simulink model "tankTry2"  (R2020a)
settings: Solver=VariableStepAuto  StartTime=0.0  StopTime=500  RelTol=1e-3
libraries: mpclib x1, simulink x1
settings Model: Creator=lydialagorga  LastModifiedBy=lydialagorga

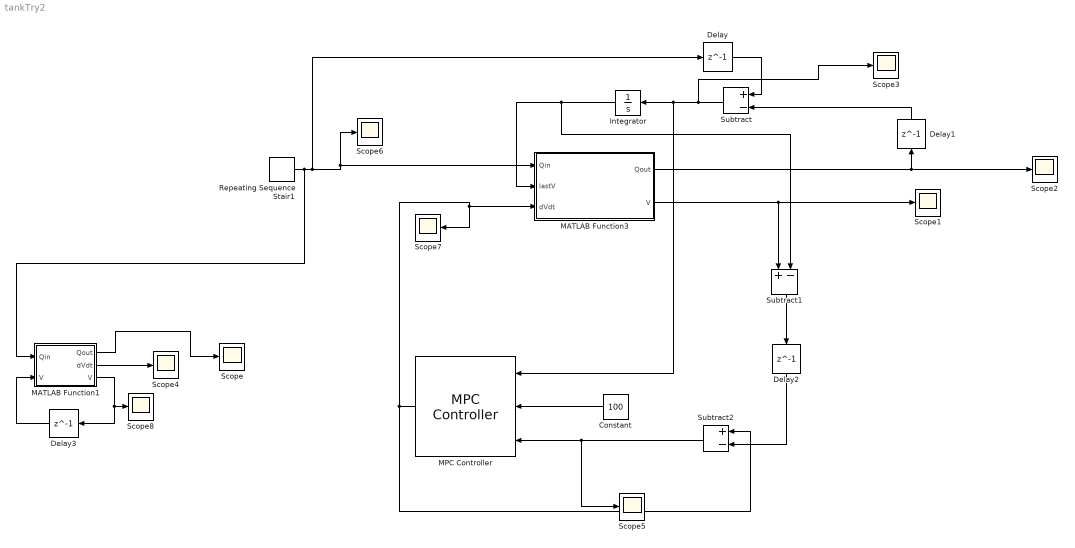
== system tankTry2 ==
  Constant : Constant  Value=100
  Delay{,1..3} (4 alike) : Delay  DelayLength=1  InitialCondition=0
  Integrator : Integrator
  MATLAB Function1 : MATLAB Function  TreatAsAtomicUnit=on
  MATLAB Function3 : MATLAB Function  TreatAsAtomicUnit=on
  MPC Controller : mpclib/MPC Controller  SCDEnableBlockLinearizationSpecification=on  mpcobj=MPCobj  is_multiple=0  enable_value=0  return_u0=off  updateMPCinCallerWorkspace=on  md_inport=on  mv_inport=off  uref_inport=off  return_cost=off  return_mvseq=off  return_qpstatus=off  return_xseq=off  return_state=off  return_ovseq=off  state_inport=off  umin_inport=off  umax_inport=off  ymin_inport=off  ymax_inport=off  cc_inport=off  ywt_inport=off  uwt_inport=off  duwt_inport=off  rhoeps_inport=off  pm_inport=off  MaximumP=10  HorizonChoice=FixedHorizon  n_ts=1  n_p=10  n_mv=1  n_md=1  n_ud=0  n_mo=1  n_uo=0  BlockDataType=double  SampleTimeInherited=off  switch_inport=off
  Repeating Sequence Stair1 : simulink/Sources/Repeating Sequence Stair  OutValues=[3 1 4 2 1]  tsamp=-1  OutMin=[]  OutMax=[]  OutDataTypeStr=double  OutputDataTypeScalingMode=double  OutDataType=fixdt(0,8)  ConRadixGroup=Best Precision: Vector-wise  OutScaling=2^-12
  Scope{,1..8} (9 alike) : Scope
  Subtract : Sum  Inputs=+-
  Subtract1 : Sum  Inputs=+-
  Subtract2 : Sum  Inputs=+-
  wires:
  MPC Controller/1 -> Scope7/1, MATLAB Function3/3(dVdt), Subtract2/1
  Repeating Sequence Stair1/1 -> MATLAB Function1/1(Qin), Delay/1, MATLAB Function3/1(Qin), Scope6/1
  Delay/1 -> Subtract/1
  Delay1/1 -> Subtract/2
  Subtract/1 -> Scope3/1, Integrator/1, MPC Controller/1
  Integrator/1 -> Subtract1/2, MATLAB Function3/2(lastV)
  MATLAB Function3/2(V) -> Scope1/1, Subtract1/1
  Subtract1/1 -> Delay2/1
  Delay2/1 -> Subtract2/2
  Subtract2/1 -> Scope5/1, MPC Controller/3
  Constant/1 -> MPC Controller/2
  MATLAB Function3/1(Qout) -> Scope2/1, Delay1/1
  MATLAB Function1/3(V) -> Scope8/1, Delay3/1
  MATLAB Function1/2(dVdt) -> Scope4/1
  MATLAB Function1/1(Qout) -> Scope/1
  Delay3/1 -> MATLAB Function1/2("V ")

== matlab function tankTry2/MATLAB Function1 ==
  data: Qin input; Qout output; V input; dVdt output; V output
function [Qout,dVdt,V] = dumbTank(Qin, V)
if Qin >= 3
   Qout = 3;
else
    Qout = Qin;
end
dVdt = Qin - Qout;
V = V + dVdt;

== matlab function tankTry2/MATLAB Function3 ==
  data: Qin input; lastV input; Qout output; dVdt input; V output
function [Qout,V]= tanky(Qin,lastV,dVdt)

V =  lastV + dVdt;
Qout = Qin-dVdt;
if Qout < 0
    Qout = 0;
end
